simulink model "base5counter"  (R2020b)
settings: Solver=VariableStepAuto  StartTime=0.0  StopTime=100  RelTol=1e-3
settings Model: EnablePacing=on  PacingRate=3  Creator=abhin  LastModifiedBy=abhin

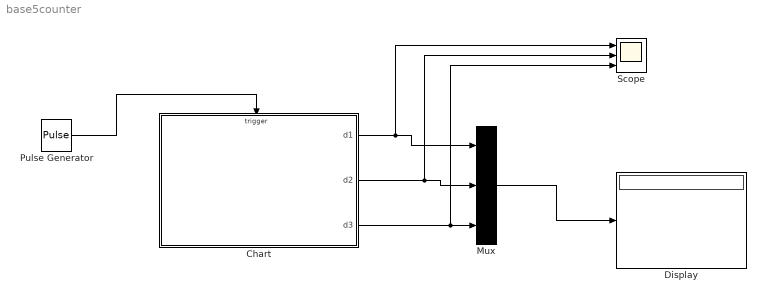
== system base5counter ==
  Chart : Stateflow chart  TreatAsAtomicUnit=on
  Display : Display
  Mux : Mux  Inputs=3
  Pulse Generator : DiscretePulseGenerator  PulseType=Time based  Period=1  PulseWidth=5
  Scope : Scope  NumInputPorts=3
  wires:
  Chart/1(d1) -> Scope/1, Mux/1
  Chart/2(d2) -> Scope/2, Mux/2
  Chart/3(d3) -> Scope/3, Mux/3
  Mux/1 -> Display/1
  Pulse Generator/1 -> Chart/Trigger

== stateflow chart base5counter/Chart ==
  state digit1 [parallel]
    settings: executionOrder=1
    state two
      en:d1=2;
    state three
      en:d1=3;
    state four
      en:d1=4;
    state zero
      en:d1=0;
    state one
      en:d1=1;
    (default) -> digit1.zero
    digit1.one -> digit1.two : inputClick
    digit1.two -> digit1.three : inputClick
    digit1.three -> digit1.four : inputClick
    digit1.zero -> digit1.one : inputClick
    digit1.four -> digit1.zero : inputClick/{digit2.inc2}
  state digit2 [parallel]
    settings: executionOrder=2
    state zero
      en:d2=0;
    state one
      en:d2=1;
    state two
      en:d2=2;
    state three
      en:d2=3;
    state four
      en:d2=4;
    digit2.zero -> digit2.one : inc2
    digit2.one -> digit2.two : inc2
    digit2.two -> digit2.three : inc2
    digit2.three -> digit2.four : inc2
    (default) -> digit2.zero
    digit2.four -> digit2.zero : inc2/{digit3.inc3}
  state digit3 [parallel]
    settings: executionOrder=3
    state zero
      en:d3=0;
    state one
      en:d3=1;
    state two
      en:d3=2;
    state three
      en:d3=3;
    state four
      en:d3=4;
    digit3.zero -> digit3.one : inc3
    digit3.one -> digit3.two : inc3
    digit3.two -> digit3.three : inc3
    digit3.three -> digit3.four : inc3
    (default) -> digit3.zero
    digit3.four -> digit3.zero : inc3
  data: d1 output; d2 output; d3 output
  events: inc2 local FUNCTION_CALL_EVENT; inc3 local FUNCTION_CALL_EVENT; inputClick input RISING_EDGE_EVENT
